simulink model "PV_cell_charactristics_Temp_2025_02_17"  (R2024a)
settings: Solver=VariableStepAuto  StartTime=0.0  StopTime=0.7  RelTol=1e-3
values from neighbouring files (symbols this model uses):
  I_75_extrapolated = interp1(x_original, I_75, x_target, 'pchip', 'extrap')    [Temperature_variation.m]
  I_matrix = cell2mat(I_new.')    [Temperature_variation.m]
  V_75_resized = interp1(x_original, V_75, x_target, 'pchip', 'extrap')    [Temperature_variation.m]    (also in V_75_resized.mat = [0.00102798669215 0.00209258422871 0.00315718182759 0.004221)
libraries: spsVoltageMeasurementLib x4, spsControlledCurrentSourceLib x2, spsControlledVoltageSourceLib x2, spsCurrentMeasurementLib x2, simulink x2, spsPVArrayLib x1, sps_lib x1
settings Model: Creator=kimiaahmadi  LastModifiedBy=kimiaahmadi

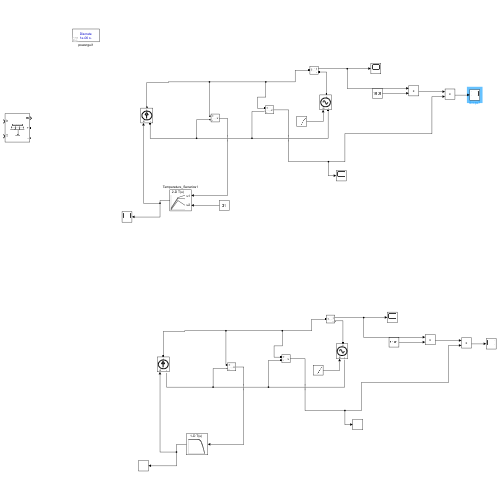
[thumbnail: Simulink's stored preview of the top-level diagram]
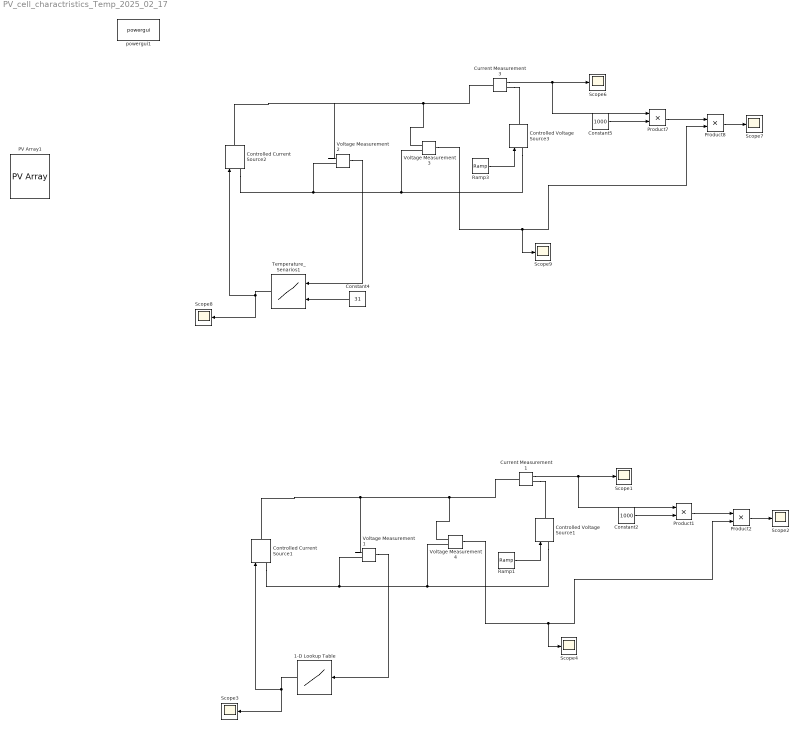
== system PV_cell_charactristics_Temp_2025_02_17 ==
  1-D Lookup Table : Lookup_n-D  NumberOfTableDimensions=1  BreakpointsForDimension1=V_75_resized  Table=I_75_extrapolated  InternalRulePriority=Speed  RndMeth=Simplest
  Constant2 : Constant  Value=1000
  Constant4 : Constant  Value=31
  Constant5 : Constant  Value=1000
  Controlled Current Source1 : spsControlledCurrentSourceLib/Controlled Current Source  Initialize=on  Source_Type=AC  Amplitude=0  Phase=0  Frequency=0  Measurements=None
  Controlled Current Source2 : spsControlledCurrentSourceLib/Controlled Current Source  Initialize=on  Source_Type=AC  Amplitude=0  Phase=0  Frequency=0  Measurements=None
  Controlled Voltage Source1 : spsControlledVoltageSourceLib/Controlled Voltage Source  Initialize=on  Source_Type=AC  Amplitude=0  Phase=0  Frequency=0  Measurements=None
  Controlled Voltage Source3 : spsControlledVoltageSourceLib/Controlled Voltage Source  Initialize=on  Source_Type=AC  Amplitude=0  Phase=0  Frequency=0  Measurements=None
  Current Measurement1 : spsCurrentMeasurementLib/Current Measurement  PhasorSimulation=off  OutputType=Complex  PSBequivalent=0
  Current Measurement3 : spsCurrentMeasurementLib/Current Measurement  PhasorSimulation=off  OutputType=Complex  PSBequivalent=0
  PV Array1 : spsPVArrayLib/PV Array  Npar=1  Nser=1  PlotType=array @ 1000 W/m2 & specified temperatures  S_vec=[75]  Temp_C_vec=[ 0:50 ]  ModuleName=User-defined  PlotWhenSelected=off  Pm=0.25  Ncell=1  Voc=0.60754  Isc=0.5737715  Vm=0.47  Im=0.53191489  beta_Voc_pc=-0.36099  alpha_Isc_pc=0.102  beta_Voc=-0.0021932  alpha_Isc=0.00058525  IL=0.57515  I0=2.136e-11  nI=0.98547  Rsh=51.3567  Rs=0.12324  RobustModel=off  RobustCellTemperature=313.3991  BAL=off  Tc=1e-6  Tfilter=5e-5
  Product{1..2,7..8} (4 alike) : Product
  Ramp1 : simulink/Sources/Ramp  slope=1  start=0  InitialOutput=0
  Ramp3 : simulink/Sources/Ramp  slope=1  start=0  InitialOutput=0
  Scope{1..4,6..9} (8 alike) : Scope
  Temperature_Senarios1 : Lookup_n-D  BreakpointsForDimension1=[0:0.001224:0.7]  BreakpointsForDimension2=[0:50]  Table=[I_matrix].'  ExtrapMethod=Clip  UseLastTableValue=on  InternalRulePriority=Speed  RndMeth=Simplest
      settings: InputPortMap=u0,u1
  Voltage Measurement{1..4} (4 alike) : spsVoltageMeasurementLib/Voltage Measurement  PhasorSimulation=off  OutputType=Complex  PSBequivalent=0
  powergui1 : sps_lib/powergui  Priority=1  SimulationMode=Discrete  SampleTime=1e-6  frequency=60  Iterations=50  frequencyindice=0  Pbase=100e6  ErrMax=1e-4  UnitsV=kV  UnitsW=MW  buscounter=0  FunctionMessages=off  echomessages=off  EnableUseOfTLC=off  CurrentSourceSwitches=off  DisableSnubberDevices=off  DisableRonSwitches=off  DisableVfSwitches=off  DisplayEquations=off  AutomaticDiscreteSolvers=off  SolverType=Tustin/Backward Euler (TBE)  Interpol=off  ExternalGateDelay=off  methode=off  Ts=100  x0status=blocks  SPID=on  SwTol=0  HookPort=off  NonlinearTolerance=1e-4  nMaxIteration=100  ContinueOnMaxIteration=off  RestoreLinks=warning  ResistiveCurrentMeasurement=off  Frange=[0:2:500]  Ylog=off  Xlog=on  ShowGrid=off  save=off  variable=ZData  structure=0  ZoomFFT=off  StartTime=0.0  cycles=1  DisplayStyle=1  fundamental=60  FreqAxis=off  MaxFrequency=1000  frequencyindicesteady=1  RmsSteady=1  display=off
  wires:
  Constant4/1 -> Temperature_Senarios1/2
  Temperature_Senarios1/1 -> Scope8/1, Controlled Current Source2/1
  Voltage Measurement2/1 -> Temperature_Senarios1/1
  Current Measurement3/1 -> Product7/1, Scope6/1
  Product7/1 -> Product8/1
  Product8/1 -> Scope7/1
  Constant5/1 -> Product7/2
  Voltage Measurement3/1 -> Scope9/1, Product8/2
  Ramp3/1 -> Controlled Voltage Source3/1
  Constant2/1 -> Product1/2
  Ramp1/1 -> Controlled Voltage Source1/1
  Voltage Measurement4/1 -> Scope4/1, Product2/2
  1-D Lookup Table/1 -> Scope3/1, Controlled Current Source1/1
  Current Measurement1/1 -> Product1/1, Scope1/1
  Product1/1 -> Product2/1
  Product2/1 -> Scope2/1
  Voltage Measurement1/1 -> 1-D Lookup Table/1
  connections:
  Voltage Measurement3/LConn2 -- Controlled Voltage Source3/LConn1 -- Controlled Current Source2/LConn1 -- Voltage Measurement2/LConn2
  Voltage Measurement3/LConn1 -- Current Measurement3/LConn1 -- Controlled Current Source2/RConn1 -- Voltage Measurement2/LConn1
  Current Measurement3/RConn1 -- Controlled Voltage Source3/RConn1
  Voltage Measurement4/LConn2 -- Controlled Voltage Source1/LConn1 -- Controlled Current Source1/LConn1 -- Voltage Measurement1/LConn2
  Voltage Measurement1/LConn1 -- Controlled Current Source1/RConn1 -- Current Measurement1/LConn1 -- Voltage Measurement4/LConn1
  Current Measurement1/RConn1 -- Controlled Voltage Source1/RConn1
